simulink model "full_system"  (R2021b)
settings: Solver=FixedStepDiscrete  StartTime=0.0  StopTime=223000  RelTol=1e-3
model workspace (MAT data in the model file):
  out_size = 0
undefined symbols (not defined in the file): betas, bias, DiscIntNeverNeededParam, mus, scale, sigmas
libraries: hdlsllib x1
(part 2 of 3)

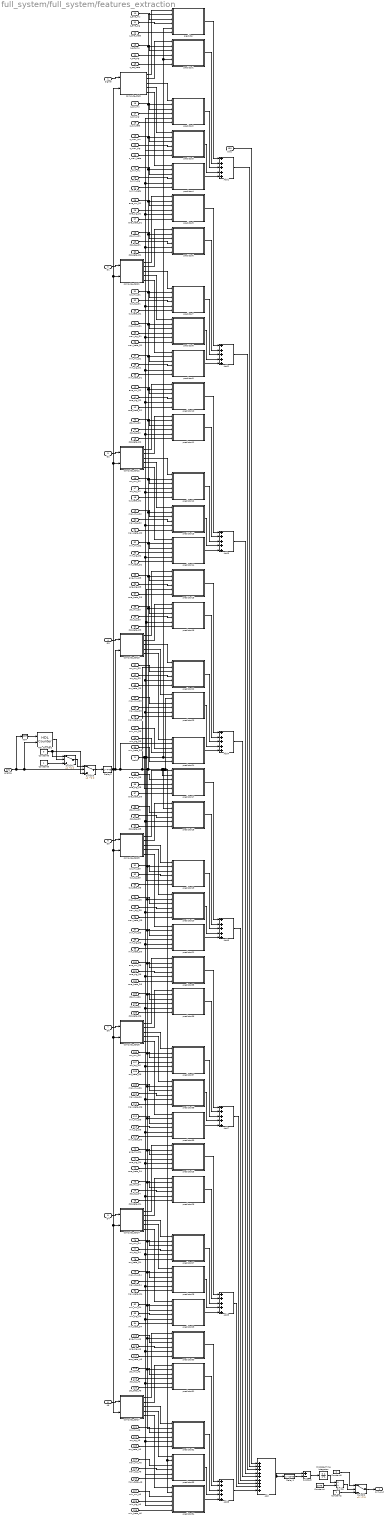
== system full_system/full_system/features_extraction ==
  Signal : Inport
  D1 : Inport  Port=2
  D2 : Inport  Port=3
  D3 : Inport  Port=4
  D4 : Inport  Port=5
  D5 : Inport  Port=6
  D6 : Inport  Port=7
  A6 : Inport  Port=8
  scale : Inport  Port=9
  s_ene_mu : Inport  Port=10
  s_ene_sig : Inport  Port=11
  s_ene_beta : Inport  Port=12
  s_act_mu : Inport  Port=13
  s_act_sig : Inport  Port=14
  s_act_beta : Inport  Port=15
  s_cur_mu : Inport  Port=16
  s_cur_sig : Inport  Port=17
  s_cur_beta : Inport  Port=18
  s_max_mu : Inport  Port=19
  s_max_sig : Inport  Port=20
  s_max_beta : Inport  Port=21
  s_min_mu : Inport  Port=22
  s_min_sig : Inport  Port=23
  s_min_beta : Inport  Port=24
  ene_mu_D1 : Inport  Port=25
  ene_sig_D1 : Inport  Port=26
  ene_beta_D1 : Inport  Port=27
  std_mu_D1 : Inport  Port=28
  std_sig_D1 : Inport  Port=29
  std_beta_D1 : Inport  Port=30
  cur_mu_D1 : Inport  Port=31
  cur_sig_D1 : Inport  Port=32
  cur_beta_D1 : Inport  Port=33
  max_mu_D1 : Inport  Port=34
  max_sig_D1 : Inport  Port=35
  max_beta_D1 : Inport  Port=36
  min_mu_D1 : Inport  Port=37
  min_sig_D1 : Inport  Port=38
  min_beta_D1 : Inport  Port=39
  ene_mu_D2 : Inport  Port=40
  ene_sig_D2 : Inport  Port=41
  ene_beta_D2 : Inport  Port=42
  std_mu_D2 : Inport  Port=43
  std_sig_D2 : Inport  Port=44
  std_beta_D2 : Inport  Port=45
  cur_mu_D2 : Inport  Port=46
  cur_sig_D2 : Inport  Port=47
  cur_beta_D2 : Inport  Port=48
  max_mu_D2 : Inport  Port=49
  max_sig_D2 : Inport  Port=50
  max_beta_D2 : Inport  Port=51
  min_mu_D2 : Inport  Port=52
  min_sig_D2 : Inport  Port=53
  min_beta_D2 : Inport  Port=54
  ene_mu_D3 : Inport  Port=55
  ene_sig_D3 : Inport  Port=56
  ene_beta_D3 : Inport  Port=57
  std_mu_D3 : Inport  Port=58
  std_sig_D3 : Inport  Port=59
  std_beta_D3 : Inport  Port=60
  cur_mu_D3 : Inport  Port=61
  cur_sig_D3 : Inport  Port=62
  cur_beta_D3 : Inport  Port=63
  max_mu_D3 : Inport  Port=64
  max_sig_D3 : Inport  Port=65
  max_beta_D3 : Inport  Port=66
  min_mu_D3 : Inport  Port=67
  min_sig_D3 : Inport  Port=68
  min_beta_D3 : Inport  Port=69
  ene_mu_D4 : Inport  Port=70
  ene_sig_D4 : Inport  Port=71
  ene_beta_D4 : Inport  Port=72
  std_mu_D4 : Inport  Port=73
  std_sig_D4 : Inport  Port=74
  std_beta_D4 : Inport  Port=75
  cur_mu_D4 : Inport  Port=76
  cur_sig_D4 : Inport  Port=77
  cur_beta_D4 : Inport  Port=78
  max_mu_D4 : Inport  Port=79
  max_sig_D4 : Inport  Port=80
  max_beta_D4 : Inport  Port=81
  min_mu_D4 : Inport  Port=82
  min_sig_D4 : Inport  Port=83
  min_beta_D4 : Inport  Port=84
  ene_mu_D5 : Inport  Port=85
  ene_sig_D5 : Inport  Port=86
  ene_beta_D5 : Inport  Port=87
  std_mu_D5 : Inport  Port=88
  std_sig_D5 : Inport  Port=89
  std_beta_D5 : Inport  Port=90
  cur_mu_D5 : Inport  Port=91
  cur_sig_D5 : Inport  Port=92
  cur_beta_D5 : Inport  Port=93
  max_mu_D5 : Inport  Port=94
  max_sig_D5 : Inport  Port=95
  max_beta_D5 : Inport  Port=96
  min_mu_D5 : Inport  Port=97
  min_sig_D5 : Inport  Port=98
  min_beta_D5 : Inport  Port=99
  ene_mu_D6 : Inport  Port=100
  ene_sig_D6 : Inport  Port=101
  ene_beta_D6 : Inport  Port=102
  std_mu_D6 : Inport  Port=103
  std_sig_D6 : Inport  Port=104
  std_beta_D6 : Inport  Port=105
  cur_mu_D6 : Inport  Port=106
  cur_sig_D6 : Inport  Port=107
  cur_beta_D6 : Inport  Port=108
  max_mu_D6 : Inport  Port=109
  max_sig_D6 : Inport  Port=110
  max_beta_D6 : Inport  Port=111
  min_mu_D6 : Inport  Port=112
  min_sig_D6 : Inport  Port=113
  min_beta_D6 : Inport  Port=114
  ene_mu_A6 : Inport  Port=115
  ene_sig_A6 : Inport  Port=116
  ene_beta_A6 : Inport  Port=117
  std_mu_A6 : Inport  Port=118
  std_sig_A6 : Inport  Port=119
  std_beta_A6 : Inport  Port=120
  cur_mu_A6 : Inport  Port=121
  cur_sig_A6 : Inport  Port=122
  cur_beta_A6 : Inport  Port=123
  max_mu_A6 : Inport  Port=124
  max_sig_A6 : Inport  Port=125
  max_beta_A6 : Inport  Port=126
  min_mu_A6 : Inport  Port=127
  min_sig_A6 : Inport  Port=128
  min_beta_A6 : Inport  Port=129
  bias : Inport  Port=130
  enable : Inport  Port=131
  Add : Sum  Inputs=+++++++++
  Add{1..8} (8 alike) : Sum  Inputs=+++++
  Constant2 : Constant  VectorParams1D=off  OutDataTypeStr=uint8  SampleTime=-1
  Constant3 : Constant  Value=0  VectorParams1D=off  OutDataTypeStr=uint8  SampleTime=-1
  Constant4 : Constant  Value=2048  VectorParams1D=off  OutDataTypeStr=uint16  SampleTime=-1
  Constant5 : Constant  VectorParams1D=off  OutDataTypeStr=boolean  SampleTime=-1
  Constant6 : Constant  Value=0  VectorParams1D=off  OutDataTypeStr=boolean  SampleTime=-1
  Delay1 : Delay  DelayLength=2049  InitialCondition=0  UseCircularBuffer=on
  Delay2 : Delay  DelayLength=449  InitialCondition=0  UseCircularBuffer=on
  Discrete-Time Integrator : DiscreteIntegrator  IntegratorMethod=Accumulation: Backward Euler  SampleTime=-1  ICPrevOutput=DiscIntNeverNeededParam  ICPrevScaledInput=DiscIntNeverNeededParam
  Divide : Product  Inputs=*/  RndMeth=Zero  SaturateOnIntegerOverflow=on  OutDataTypeStr=Inherit: Same as first input
  HDL Counter1 : hdlsllib/Sources/HDL Counter  CountType=Count limited  CountInit=0  CountStep=1  CountMax=511  CountFromType=Initial value  CountFrom=0  CountResetPort=on  CountLoadPort=off  CountEnbPort=on  CountDirPort=off  CountHitOutputPort=off  CountDataType=Unsigned  CountWordLen=9  CountFracLen=0  CountSampTime=1
  NOT : Logic  Operator=NOT  IconShape=distinctive  AllPortsSameDT=off  OutDataTypeStr=boolean
  Subtract : Sum  Inputs=+-
  Switch1 : Switch  Criteria=u2 ~= 0
  Switch2 : Switch
  Switch3 : Switch  Criteria=u2 ~= 0
  compute_stats : Subsystem
  compute_stats1 : Subsystem
  compute_stats2 : Subsystem
  compute_stats3 : Subsystem
  compute_stats4 : Subsystem
  compute_stats5 : Subsystem
  compute_stats6 : Subsystem
  compute_stats7 : Subsystem
  predictor{,1..39} (40 alike) : Subsystem  ReferencedSubsystem=predictor_2021b
  svm_out : Outport
  wires:
  cur_sig_D4/1 -> predictor27/4
  predictor1/1 -> Add1/2
  HDL Counter1/1 -> Switch1/2
  ene_mu_D1/1 -> predictor5/3
  Constant5/1 -> Switch1/3
  compute_stats1/1(energy) -> predictor5/1
  predictor11/1 -> Add3/2
  Delay1/1 -> Subtract/2
  compute_stats2/2(std) -> predictor11/1
  predictor29/1 -> Add5/5
  Constant4/1 -> Divide/2
  std_sig_A6/1 -> predictor31/4
  Switch1/1 -> Switch3/1  "trigger"
  predictor3/1 -> Add1/4
  Add1/1 -> Add/2
  Add3/1 -> Add/4
  NOT/1 -> HDL Counter1/1
  s_ene_sig/1 -> predictor/4
  Switch3/1 -> Delay2/1  "trigger"
  compute_stats6/1(energy) -> predictor35/1
  Discrete-Time Integrator/1 -> Divide/1
  compute_stats5/3(curve_l) -> predictor19/1
  predictor13/1 -> Add3/4
  Divide/1 -> Switch2/2  "average"
  predictor18/1 -> Add6/2
  predictor39/1 -> Add7/5
  Switch2/1 -> svm_out/1  "out"
  Subtract/1 -> Discrete-Time Integrator/1
  predictor5/1 -> Add2/1
  predictor23/1 -> Add4/4
  bias/1 -> Add/1
  Add2/1 -> Add/3
  predictor14/1 -> Add3/5
  std_sig_D3/1 -> predictor16/4
  predictor31/1 -> Add8/2
  max_mu_D2/1 -> predictor13/3
  Add4/1 -> Add/5
  std_mu_D2/1 -> predictor11/3
  Add5/1 -> Add/8
  max_mu_D3/1 -> predictor23/3
  predictor32/1 -> Add8/3
  Add6/1 -> Add/6
  Add7/1 -> Add/7
  predictor22/1 -> Add4/3
  Add8/1 -> Add/9
  predictor33/1 -> Add8/4
  ene_sig_A6/1 -> predictor30/4
  predictor6/1 -> Add2/2
  predictor10/1 -> Add3/1
  compute_stats7/2(std) -> predictor31/1
  predictor30/1 -> Add8/1
  predictor34/1 -> Add8/5
  predictor37/1 -> Add7/3
  predictor36/1 -> Add7/2
  predictor38/1 -> Add7/4
  predictor35/1 -> Add7/1
  min_mu_D5/1 -> predictor21/3
  predictor19/1 -> Add6/3
  predictor20/1 -> Add6/4
  max_beta_A6/1 -> predictor33/6
  predictor17/1 -> Add6/1
  compute_stats6/3(curve_l) -> predictor37/1
  predictor21/1 -> Add6/5
  predictor27/1 -> Add5/3
  predictor26/1 -> Add5/2
  predictor28/1 -> Add5/4
  predictor8/1 -> Add2/4
  predictor25/1 -> Add5/1
  predictor16/1 -> Add4/2
  predictor12/1 -> Add3/3
  predictor15/1 -> Add4/1
  Constant2/1 -> Switch2/3
  min_mu_D1/1 -> predictor9/3
  predictor/1 -> Add1/1
  predictor24/1 -> Add4/5
  ene_mu_D2/1 -> predictor10/3
  predictor7/1 -> Add2/3
  predictor9/1 -> Add2/5
  predictor4/1 -> Add1/5
  ene_sig_D4/1 -> predictor25/4
  predictor2/1 -> Add1/3
  min_beta_A6/1 -> predictor34/6
  cur_sig_A6/1 -> predictor32/4
  cur_mu_A6/1 -> predictor32/3
  max_mu_A6/1 -> predictor33/3
  min_mu_A6/1 -> predictor34/3
  std_mu_A6/1 -> predictor31/3
  cur_beta_A6/1 -> predictor32/6
  ene_beta_A6/1 -> predictor30/6
  std_beta_A6/1 -> predictor31/6
  min_sig_A6/1 -> predictor34/4
  ene_mu_A6/1 -> predictor30/3
  max_sig_A6/1 -> predictor33/4
  min_beta_D6/1 -> predictor39/6
  max_beta_D6/1 -> predictor38/6
  cur_sig_D6/1 -> predictor37/4
  cur_mu_D6/1 -> predictor37/3
  max_mu_D6/1 -> predictor38/3
  ene_sig_D6/1 -> predictor35/4
  min_mu_D6/1 -> predictor39/3
  std_sig_D6/1 -> predictor36/4
  std_mu_D6/1 -> predictor36/3
  cur_beta_D6/1 -> predictor37/6
  ene_beta_D6/1 -> predictor35/6
  std_beta_D6/1 -> predictor36/6
  min_sig_D6/1 -> predictor39/4
  ene_mu_D6/1 -> predictor35/3
  max_sig_D6/1 -> predictor38/4
  min_beta_D5/1 -> predictor21/6
  max_beta_D5/1 -> predictor20/6
  cur_sig_D5/1 -> predictor19/4
  cur_mu_D5/1 -> predictor19/3
  max_mu_D5/1 -> predictor20/3
  ene_sig_D5/1 -> predictor17/4
  std_sig_D5/1 -> predictor18/4
  std_mu_D5/1 -> predictor18/3
  cur_beta_D5/1 -> predictor19/6
  ene_beta_D5/1 -> predictor17/6
  std_beta_D5/1 -> predictor18/6
  min_sig_D5/1 -> predictor21/4
  ene_mu_D5/1 -> predictor17/3
  max_sig_D5/1 -> predictor20/4
  min_beta_D4/1 -> predictor29/6
  max_beta_D4/1 -> predictor28/6
  cur_mu_D4/1 -> predictor27/3
  Constant6/1 -> Switch1/1, Switch3/3
  max_mu_D4/1 -> predictor28/3
  min_mu_D4/1 -> predictor29/3
  std_sig_D4/1 -> predictor26/4
  std_mu_D4/1 -> predictor26/3
  cur_beta_D4/1 -> predictor27/6
  ene_beta_D4/1 -> predictor25/6
  std_beta_D4/1 -> predictor26/6
  min_sig_D4/1 -> predictor29/4
  ene_mu_D4/1 -> predictor25/3
  max_sig_D4/1 -> predictor28/4
  min_beta_D3/1 -> predictor24/6
  max_beta_D3/1 -> predictor23/6
  compute_stats5/5(min) -> predictor21/1
  cur_sig_D3/1 -> predictor22/4
  cur_mu_D3/1 -> predictor22/3
  ene_sig_D3/1 -> predictor15/4
  min_mu_D3/1 -> predictor24/3
  std_mu_D3/1 -> predictor16/3
  cur_beta_D3/1 -> predictor22/6
  ene_beta_D3/1 -> predictor15/6
  std_beta_D3/1 -> predictor16/6
  min_sig_D3/1 -> predictor24/4
  compute_stats6/2(std) -> predictor36/1
  ene_mu_D3/1 -> predictor15/3
  max_sig_D3/1 -> predictor23/4
  min_beta_D2/1 -> predictor14/6
  D3/1 -> compute_stats3/1(in)
  max_beta_D2/1 -> predictor13/6
  cur_sig_D2/1 -> predictor12/4
  cur_mu_D2/1 -> predictor12/3
  ene_sig_D2/1 -> predictor10/4
  compute_stats7/1(energy) -> predictor30/1
  min_mu_D2/1 -> predictor14/3
  std_sig_D2/1 -> predictor11/4
  cur_beta_D2/1 -> predictor12/6
  ene_beta_D2/1 -> predictor10/6
  std_beta_D2/1 -> predictor11/6
  min_sig_D2/1 -> predictor14/4
  max_sig_D2/1 -> predictor13/4
  min_beta_D1/1 -> predictor9/6
  max_beta_D1/1 -> predictor8/6
  cur_sig_D1/1 -> predictor7/4
  cur_mu_D1/1 -> predictor7/3
  max_mu_D1/1 -> predictor8/3
  ene_sig_D1/1 -> predictor5/4
  std_sig_D1/1 -> predictor6/4
  std_mu_D1/1 -> predictor6/3
  cur_beta_D1/1 -> predictor7/6
  ene_beta_D1/1 -> predictor5/6
  std_beta_D1/1 -> predictor6/6
  min_sig_D1/1 -> predictor9/4
  max_sig_D1/1 -> predictor8/4
  s_min_beta/1 -> predictor4/6
  s_min_mu/1 -> predictor4/3
  s_min_sig/1 -> predictor4/4
  s_max_beta/1 -> predictor3/6
  s_max_mu/1 -> predictor3/3
  s_max_sig/1 -> predictor3/4
  s_cur_beta/1 -> predictor2/6
  s_cur_mu/1 -> predictor2/3
  s_cur_sig/1 -> predictor2/4
  s_act_beta/1 -> predictor1/6
  s_act_mu/1 -> predictor1/3
  s_act_sig/1 -> predictor1/4
  s_ene_beta/1 -> predictor/6
  s_ene_mu/1 -> predictor/3
  compute_stats3/5(min) -> predictor24/1
  compute_stats7/5(min) -> predictor34/1
  compute_stats7/4(max) -> predictor33/1
  compute_stats7/3(curve_l) -> predictor32/1
  Delay2/1 -> compute_stats7/2(trigger), compute_stats4/2(trigger), compute_stats6/2(trigger), compute_stats5/2(trigger), predictor32/2, predictor31/2, predictor30/2, predictor29/2, predictor28/2, predictor27/2, predictor26/2, predictor25/2, predictor39/2, predictor38/2, predictor37/2, predictor36/2, predictor35/2, predictor21/2, predictor20/2, predictor19/2, predictor33/2, predictor34/2, predictor23/2, predictor18/2, predictor17/2, predictor1/2, predictor/2, predictor2/2, predictor3/2, predictor4/2, predictor5/2, predictor6/2, predictor7/2, predictor8/2, predictor9/2, predictor10/2, predictor11/2, predictor12/2, predictor13/2, predictor14/2, predictor15/2, predictor16/2, predictor22/2, predictor24/2, compute_stats3/2(trigger), compute_stats1/2(trigger), compute_stats/2(trigger), compute_stats2/2(trigger)  "trigger"
  compute_stats6/5(min) -> predictor39/1
  compute_stats6/4(max) -> predictor38/1
  compute_stats5/4(max) -> predictor20/1
  compute_stats5/2(std) -> predictor18/1
  compute_stats5/1(energy) -> predictor17/1
  compute_stats4/5(min) -> predictor29/1
  compute_stats4/4(max) -> predictor28/1
  compute_stats4/3(curve_l) -> predictor27/1
  compute_stats4/2(std) -> predictor26/1
  compute_stats4/1(energy) -> predictor25/1
  compute_stats3/4(max) -> predictor23/1
  compute_stats3/3(curve_l) -> predictor22/1
  compute_stats3/2(std) -> predictor16/1
  compute_stats3/1(energy) -> predictor15/1
  compute_stats2/5(min) -> predictor14/1
  compute_stats2/4(max) -> predictor13/1
  compute_stats2/3(curve_l) -> predictor12/1
  compute_stats2/1(energy) -> predictor10/1
  compute_stats1/5(min) -> predictor9/1
  compute_stats1/4(max) -> predictor8/1
  compute_stats1/3(curve_l) -> predictor7/1
  compute_stats1/2(std) -> predictor6/1
  compute_stats/5(min) -> predictor4/1
  compute_stats/4(max) -> predictor3/1
  compute_stats/3(curve_l) -> predictor2/1
  compute_stats/2(activity) -> predictor1/1
  compute_stats/1(energy) -> predictor/1
  Add/1 -> Delay1/1, Subtract/1  "in"
  Constant3/1 -> Switch2/1
  A6/1 -> compute_stats7/1(in)
  D6/1 -> compute_stats6/1(in)
  D5/1 -> compute_stats5/1(in)
  D4/1 -> compute_stats4/1(in)
  D2/1 -> compute_stats2/1(in)
  D1/1 -> compute_stats1/1(in)
  Signal/1 -> compute_stats/1(in)  "signal"
  enable/1 -> HDL Counter1/2, Switch3/2, NOT/1
  scale/1 -> predictor34/5, predictor32/5, predictor31/5, predictor30/5, predictor29/5, predictor28/5, predictor27/5, predictor26/5, predictor25/5, predictor33/5, predictor39/5, predictor38/5, predictor37/5, predictor36/5, predictor35/5, predictor21/5, predictor20/5, predictor18/5, predictor1/5, predictor/5, predictor24/5, predictor16/5, predictor15/5, predictor19/5, predictor4/5, predictor3/5, predictor5/5, predictor6/5, predictor7/5, predictor8/5, predictor9/5, predictor10/5, predictor11/5, predictor12/5, predictor13/5, predictor14/5, predictor22/5, predictor23/5, predictor2/5, predictor17/5

== system full_system/full_system/4_level_dwt/1_level_dwt ==
  s_in : Inport
  enable : Inport  Port=2
  Constant : Constant  Value=0  OutDataTypeStr=Inherit: Inherit via back propagation  SampleTime=-1
  Discrete FIR Filter : DiscreteFir  CoefSource=Input port
      settings: InputPortMap=u0,u1
  Discrete FIR Filter1 : DiscreteFir  CoefSource=Input port
      settings: InputPortMap=u0,u1
  Downsample : DownSample  phase=1  RateOptions=Allow multirate processing
  Downsample1 : DownSample  phase=1  RateOptions=Allow multirate processing
  RT2 : RateTransition  OutPortSampleTime=2
  Switch : Switch  Criteria=u2 > Threshold
  Switch1 : Switch  Criteria=u2 > Threshold
  db4 scaling : Constant  Value="[-0.0106    0.0329    0.0308   -0.1870   -0.0280    0.6309    0.7148    0.2304]"  OutDataTypeStr=Inherit: Inherit via back propagation  SampleTime=-1
  db4 wavelet : Constant  Value="[-0.2304    0.7148   -0.6309   -0.0280    0.1870    0.0308   -0.0329   -0.0106]"  OutDataTypeStr=Inherit: Inherit via back propagation  SampleTime=-1
  D : Outport
  A : Outport  Port=2
  wires:
  db4 wavelet/1 -> Discrete FIR Filter/2
  s_in/1 -> Discrete FIR Filter1/1, Discrete FIR Filter/1
  db4 scaling/1 -> Discrete FIR Filter1/2
  Constant/1 -> Switch/3, Switch1/3
  Discrete FIR Filter/1 -> Downsample/1
  Discrete FIR Filter1/1 -> Downsample1/1
  Switch1/1 -> A/1
  Switch/1 -> D/1
  Downsample/1 -> Switch/1
  Downsample1/1 -> Switch1/1
  enable/1 -> RT2/1
  RT2/1 -> Switch/2, Switch1/2

== system full_system/full_system/4_level_dwt/1_level_dwt1 ==
  s_in : Inport
  enable : Inport  Port=2
  Constant : Constant  Value=0  OutDataTypeStr=Inherit: Inherit via back propagation  SampleTime=-1
  Discrete FIR Filter : DiscreteFir  CoefSource=Input port
      settings: InputPortMap=u0,u1
  Discrete FIR Filter1 : DiscreteFir  CoefSource=Input port
      settings: InputPortMap=u0,u1
  Downsample : DownSample  phase=1  RateOptions=Allow multirate processing
  Downsample1 : DownSample  phase=1  RateOptions=Allow multirate processing
  RT2 : RateTransition  OutPortSampleTime=4
  Switch : Switch  Criteria=u2 > Threshold
  Switch1 : Switch  Criteria=u2 > Threshold
  db4 scaling : Constant  Value="[-0.0106    0.0329    0.0308   -0.1870   -0.0280    0.6309    0.7148    0.2304]"  OutDataTypeStr=Inherit: Inherit via back propagation  SampleTime=-1
  db4 wavelet : Constant  Value="[-0.2304    0.7148   -0.6309   -0.0280    0.1870    0.0308   -0.0329   -0.0106]"  OutDataTypeStr=Inherit: Inherit via back propagation  SampleTime=-1
  D : Outport
  A : Outport  Port=2
  wires:
  db4 wavelet/1 -> Discrete FIR Filter/2
  s_in/1 -> Discrete FIR Filter1/1, Discrete FIR Filter/1
  db4 scaling/1 -> Discrete FIR Filter1/2
  Constant/1 -> Switch/3, Switch1/3
  Discrete FIR Filter/1 -> Downsample/1
  Discrete FIR Filter1/1 -> Downsample1/1
  Switch1/1 -> A/1
  Switch/1 -> D/1
  Downsample/1 -> Switch/1
  Downsample1/1 -> Switch1/1
  enable/1 -> RT2/1
  RT2/1 -> Switch/2, Switch1/2

== system full_system/full_system/4_level_dwt/1_level_dwt2 ==
  s_in : Inport
  enable : Inport  Port=2
  Constant : Constant  Value=0  OutDataTypeStr=Inherit: Inherit via back propagation  SampleTime=-1
  Discrete FIR Filter : DiscreteFir  CoefSource=Input port
      settings: InputPortMap=u0,u1
  Discrete FIR Filter1 : DiscreteFir  CoefSource=Input port
      settings: InputPortMap=u0,u1
  Downsample : DownSample  phase=1  RateOptions=Allow multirate processing
  Downsample1 : DownSample  phase=1  RateOptions=Allow multirate processing
  RT2 : RateTransition  OutPortSampleTime=8
  Switch : Switch  Criteria=u2 > Threshold
  Switch1 : Switch  Criteria=u2 > Threshold
  db4 scaling : Constant  Value="[-0.0106    0.0329    0.0308   -0.1870   -0.0280    0.6309    0.7148    0.2304]"  OutDataTypeStr=Inherit: Inherit via back propagation  SampleTime=-1
  db4 wavelet : Constant  Value="[-0.2304    0.7148   -0.6309   -0.0280    0.1870    0.0308   -0.0329   -0.0106]"  OutDataTypeStr=Inherit: Inherit via back propagation  SampleTime=-1
  D : Outport
  A : Outport  Port=2
  wires:
  db4 wavelet/1 -> Discrete FIR Filter/2
  s_in/1 -> Discrete FIR Filter1/1, Discrete FIR Filter/1
  db4 scaling/1 -> Discrete FIR Filter1/2
  Constant/1 -> Switch/3, Switch1/3
  Discrete FIR Filter/1 -> Downsample/1
  Discrete FIR Filter1/1 -> Downsample1/1
  Switch1/1 -> A/1
  Switch/1 -> D/1
  Downsample/1 -> Switch/1
  Downsample1/1 -> Switch1/1
  enable/1 -> RT2/1
  RT2/1 -> Switch/2, Switch1/2

== system full_system/full_system/4_level_dwt/1_level_dwt3 ==
  s_in : Inport
  enable : Inport  Port=2
  Constant : Constant  Value=0  OutDataTypeStr=Inherit: Inherit via back propagation  SampleTime=-1
  Discrete FIR Filter : DiscreteFir  CoefSource=Input port
      settings: InputPortMap=u0,u1
  Discrete FIR Filter1 : DiscreteFir  CoefSource=Input port
      settings: InputPortMap=u0,u1
  Downsample : DownSample  phase=1  RateOptions=Allow multirate processing
  Downsample1 : DownSample  phase=1  RateOptions=Allow multirate processing
  RT2 : RateTransition  OutPortSampleTime=16
  Switch : Switch  Criteria=u2 > Threshold
  Switch1 : Switch  Criteria=u2 > Threshold
  db4 scaling : Constant  Value="[-0.0106    0.0329    0.0308   -0.1870   -0.0280    0.6309    0.7148    0.2304]"  OutDataTypeStr=Inherit: Inherit via back propagation  SampleTime=-1
  db4 wavelet : Constant  Value="[-0.2304    0.7148   -0.6309   -0.0280    0.1870    0.0308   -0.0329   -0.0106]"  OutDataTypeStr=Inherit: Inherit via back propagation  SampleTime=-1
  D : Outport
  A : Outport  Port=2
  wires:
  db4 wavelet/1 -> Discrete FIR Filter/2
  s_in/1 -> Discrete FIR Filter1/1, Discrete FIR Filter/1
  db4 scaling/1 -> Discrete FIR Filter1/2
  Constant/1 -> Switch/3, Switch1/3
  Discrete FIR Filter/1 -> Downsample/1
  Switch1/1 -> A/1
  Switch/1 -> D/1
  Downsample/1 -> Switch/1
  Downsample1/1 -> Switch1/1
  enable/1 -> RT2/1
  RT2/1 -> Switch/2, Switch1/2
  Discrete FIR Filter1/1 -> Downsample1/1

== system full_system/full_system/4_level_dwt/1_level_dwt4 ==
  s_in : Inport
  enable : Inport  Port=2
  Constant : Constant  Value=0  OutDataTypeStr=Inherit: Inherit via back propagation  SampleTime=-1
  Discrete FIR Filter : DiscreteFir  CoefSource=Input port
      settings: InputPortMap=u0,u1
  Discrete FIR Filter1 : DiscreteFir  CoefSource=Input port
      settings: InputPortMap=u0,u1
  Downsample : DownSample  phase=1  RateOptions=Allow multirate processing
  Downsample1 : DownSample  phase=1  RateOptions=Allow multirate processing
  RT2 : RateTransition  OutPortSampleTime=32
  Switch : Switch  Criteria=u2 > Threshold
  Switch1 : Switch  Criteria=u2 > Threshold
  db4 scaling : Constant  Value="[-0.0106    0.0329    0.0308   -0.1870   -0.0280    0.6309    0.7148    0.2304]"  OutDataTypeStr=Inherit: Inherit via back propagation  SampleTime=-1
  db4 wavelet : Constant  Value="[-0.2304    0.7148   -0.6309   -0.0280    0.1870    0.0308   -0.0329   -0.0106]"  OutDataTypeStr=Inherit: Inherit via back propagation  SampleTime=-1
  D : Outport
  A : Outport  Port=2
  wires:
  db4 wavelet/1 -> Discrete FIR Filter/2
  s_in/1 -> Discrete FIR Filter1/1, Discrete FIR Filter/1
  db4 scaling/1 -> Discrete FIR Filter1/2
  Constant/1 -> Switch/3, Switch1/3
  Discrete FIR Filter/1 -> Downsample/1
  Switch1/1 -> A/1
  Switch/1 -> D/1
  Downsample/1 -> Switch/1
  Downsample1/1 -> Switch1/1
  enable/1 -> RT2/1
  RT2/1 -> Switch/2, Switch1/2
  Discrete FIR Filter1/1 -> Downsample1/1

== system full_system/full_system/4_level_dwt/1_level_dwt5 ==
  s_in : Inport
  enable : Inport  Port=2
  Constant : Constant  Value=0  OutDataTypeStr=Inherit: Inherit via back propagation  SampleTime=-1
  Discrete FIR Filter : DiscreteFir  CoefSource=Input port
      settings: InputPortMap=u0,u1
  Discrete FIR Filter1 : DiscreteFir  CoefSource=Input port
      settings: InputPortMap=u0,u1
  Downsample : DownSample  phase=1  RateOptions=Allow multirate processing
  Downsample1 : DownSample  phase=1  RateOptions=Allow multirate processing
  RT2 : RateTransition  OutPortSampleTime=64
  Switch : Switch  Criteria=u2 > Threshold
  Switch1 : Switch  Criteria=u2 > Threshold
  db4 scaling : Constant  Value="[-0.0106    0.0329    0.0308   -0.1870   -0.0280    0.6309    0.7148    0.2304]"  OutDataTypeStr=Inherit: Inherit via back propagation  SampleTime=-1
  db4 wavelet : Constant  Value="[-0.2304    0.7148   -0.6309   -0.0280    0.1870    0.0308   -0.0329   -0.0106]"  OutDataTypeStr=Inherit: Inherit via back propagation  SampleTime=-1
  D : Outport
  A : Outport  Port=2
  wires:
  db4 wavelet/1 -> Discrete FIR Filter/2
  s_in/1 -> Discrete FIR Filter1/1, Discrete FIR Filter/1
  db4 scaling/1 -> Discrete FIR Filter1/2
  Constant/1 -> Switch/3, Switch1/3
  Discrete FIR Filter/1 -> Downsample/1
  Switch1/1 -> A/1
  Switch/1 -> D/1
  Downsample/1 -> Switch/1
  Downsample1/1 -> Switch1/1
  enable/1 -> RT2/1
  RT2/1 -> Switch/2, Switch1/2
  Discrete FIR Filter1/1 -> Downsample1/1

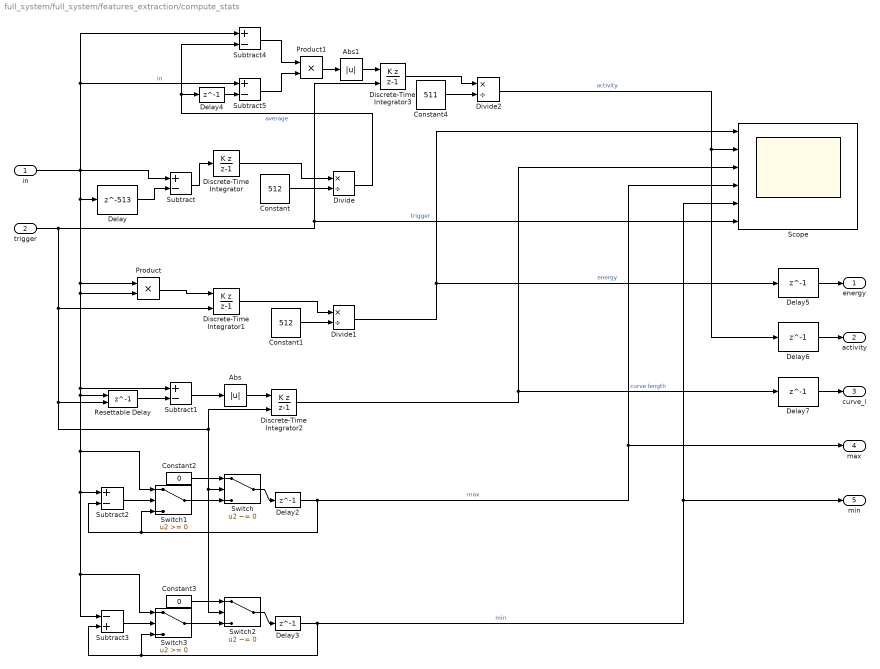
== system full_system/full_system/features_extraction/compute_stats ==
  in : Inport
  trigger : Inport  Port=2
  Abs : Abs
  Abs1 : Abs
  Constant : Constant  Value=512  VectorParams1D=off  OutDataTypeStr=uint16  SampleTime=-1
  Constant1 : Constant  Value=512  VectorParams1D=off  OutDataTypeStr=uint16  SampleTime=-1
  Constant2 : Constant  Value=0  VectorParams1D=off  OutDataTypeStr=uint8  SampleTime=-1
  Constant3 : Constant  Value=0  VectorParams1D=off  OutDataTypeStr=uint8  SampleTime=-1
  Constant4 : Constant  Value=511  VectorParams1D=off  OutDataTypeStr=uint16  SampleTime=-1
  Delay : Delay  DelayLength=513  InitialCondition=0  UseCircularBuffer=on
  Delay{2..7} (6 alike) : Delay  DelayLength=1  InitialCondition=0  UseCircularBuffer=on
  Discrete-Time Integrator : DiscreteIntegrator  IntegratorMethod=Accumulation: Backward Euler  SampleTime=-1  ICPrevOutput=DiscIntNeverNeededParam  ICPrevScaledInput=DiscIntNeverNeededParam
  Discrete-Time Integrator1 : DiscreteIntegrator  IntegratorMethod=Accumulation: Backward Euler  ExternalReset=rising  SampleTime=-1  ICPrevOutput=DiscIntNeverNeededParam  ICPrevScaledInput=DiscIntNeverNeededParam
  Discrete-Time Integrator2 : DiscreteIntegrator  IntegratorMethod=Accumulation: Backward Euler  ExternalReset=rising  SampleTime=-1  ICPrevOutput=DiscIntNeverNeededParam  ICPrevScaledInput=DiscIntNeverNeededParam
  Discrete-Time Integrator3 : DiscreteIntegrator  IntegratorMethod=Accumulation: Backward Euler  ExternalReset=rising  SampleTime=-1  ICPrevOutput=DiscIntNeverNeededParam  ICPrevScaledInput=DiscIntNeverNeededParam
  Divide : Product  Inputs=*/  RndMeth=Zero  SaturateOnIntegerOverflow=on  OutDataTypeStr=Inherit: Same as first input
  Divide1 : Product  Inputs=*/  RndMeth=Zero  SaturateOnIntegerOverflow=on
  Divide2 : Product  Inputs=*/  RndMeth=Zero  SaturateOnIntegerOverflow=on
  Product : Product
  Product1 : Product
  Resettable Delay : Delay  DelayLength=1  ExternalReset=Level
      settings: InputPortMap=u0,r5
  Scope : Scope  NumInputPorts=6
  Subtract{,1..2,4..5} (5 alike) : Sum  Inputs=+-
  Subtract3 : Sum  Inputs=-+
  Switch : Switch  Criteria=u2 ~= 0
  Switch1 : Switch  OutDataTypeStr=Inherit: Same as first input
  Switch2 : Switch  Criteria=u2 ~= 0
  Switch3 : Switch  OutDataTypeStr=Inherit: Same as first input
  energy : Outport
  activity : Outport  Port=2
  curve_l : Outport  Port=3
  max : Outport  Port=4
  min : Outport  Port=5
  wires:
  Constant/1 -> Divide/2
  Subtract/1 -> Discrete-Time Integrator/1
  Delay/1 -> Subtract/2
  Product/1 -> Discrete-Time Integrator1/1
  Constant1/1 -> Divide1/2
  Discrete-Time Integrator1/1 -> Divide1/1
  Resettable Delay/1 -> Subtract1/2
  Subtract1/1 -> Abs/1
  Abs/1 -> Discrete-Time Integrator2/1
  Discrete-Time Integrator2/1 -> Delay7/1, Scope/3  "curve length"
  Constant2/1 -> Switch/1
  Subtract2/1 -> Switch1/2
  Delay2/1 -> max/1, Scope/4, Switch1/3, Subtract2/2  "max"
  Switch/1 -> Delay2/1
  Switch1/1 -> Switch/3
  Constant3/1 -> Switch2/1
  Switch2/1 -> Delay3/1
  Switch3/1 -> Switch2/3
  Subtract3/1 -> Switch3/2
  Delay3/1 -> min/1, Scope/5, Switch3/3, Subtract3/2  "min"
  Delay4/1 -> Subtract5/2
  Subtract4/1 -> Product1/1
  Subtract5/1 -> Product1/2
  Constant4/1 -> Divide2/2
  Discrete-Time Integrator3/1 -> Divide2/1
  Divide/1 -> Subtract4/2, Delay4/1  "average"
  Discrete-Time Integrator/1 -> Divide/1
  Divide2/1 -> Scope/2, Delay6/1  "activity"
  Product1/1 -> Abs1/1
  Abs1/1 -> Discrete-Time Integrator3/1
  Delay5/1 -> energy/1
  Delay6/1 -> activity/1
  Delay7/1 -> curve_l/1
  Divide1/1 -> Scope/1, Delay5/1  "energy"
  in/1 -> Delay/1, Product/1, Resettable Delay/1, Switch1/1, Switch3/1, Subtract3/1, Subtract2/1, Subtract1/1, Product/2, Subtract4/1, Subtract5/1, Subtract/1  "in"
  trigger/1 -> Discrete-Time Integrator3/2, Scope/6, Discrete-Time Integrator1/2, Resettable Delay/2, Discrete-Time Integrator2/2, Switch2/2, Switch/2  "trigger"

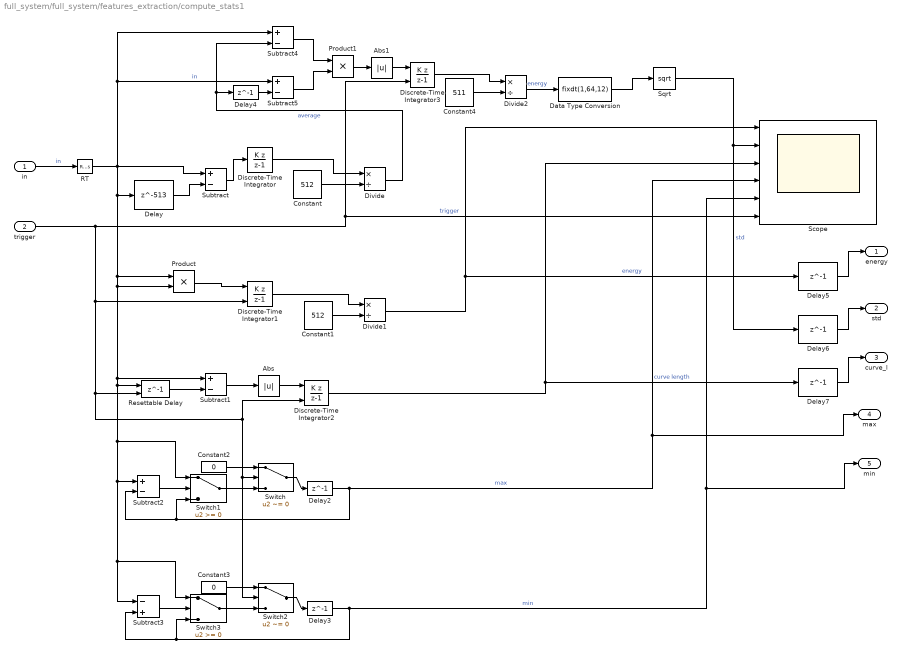
== system full_system/full_system/features_extraction/compute_stats1 ==
  in : Inport
  trigger : Inport  Port=2
  Abs : Abs
  Abs1 : Abs
  Constant : Constant  Value=512  VectorParams1D=off  OutDataTypeStr=uint16  SampleTime=-1
  Constant1 : Constant  Value=512  VectorParams1D=off  OutDataTypeStr=uint16  SampleTime=-1
  Constant2 : Constant  Value=0  VectorParams1D=off  OutDataTypeStr=uint8  SampleTime=-1
  Constant3 : Constant  Value=0  VectorParams1D=off  OutDataTypeStr=uint8  SampleTime=-1
  Constant4 : Constant  Value=511  VectorParams1D=off  OutDataTypeStr=uint16  SampleTime=-1
  Data Type Conversion : DataTypeConversion  OutMax=2  OutDataTypeStr=fixdt(1,64,12)
  Delay : Delay  DelayLength=513  InitialCondition=0  UseCircularBuffer=on
  Delay{2..7} (6 alike) : Delay  DelayLength=1  InitialCondition=0  UseCircularBuffer=on
  Discrete-Time Integrator : DiscreteIntegrator  IntegratorMethod=Accumulation: Backward Euler  SampleTime=-1  ICPrevOutput=DiscIntNeverNeededParam  ICPrevScaledInput=DiscIntNeverNeededParam
  Discrete-Time Integrator1 : DiscreteIntegrator  IntegratorMethod=Accumulation: Backward Euler  ExternalReset=rising  SampleTime=-1  ICPrevOutput=DiscIntNeverNeededParam  ICPrevScaledInput=DiscIntNeverNeededParam
  Discrete-Time Integrator2 : DiscreteIntegrator  IntegratorMethod=Accumulation: Backward Euler  ExternalReset=rising  SampleTime=-1  ICPrevOutput=DiscIntNeverNeededParam  ICPrevScaledInput=DiscIntNeverNeededParam
  Discrete-Time Integrator3 : DiscreteIntegrator  IntegratorMethod=Accumulation: Backward Euler  ExternalReset=rising  SampleTime=-1  ICPrevOutput=DiscIntNeverNeededParam  ICPrevScaledInput=DiscIntNeverNeededParam
  Divide : Product  Inputs=*/  RndMeth=Zero  SaturateOnIntegerOverflow=on  OutDataTypeStr=Inherit: Same as first input
  Divide1 : Product  Inputs=*/  RndMeth=Zero  SaturateOnIntegerOverflow=on
  Divide2 : Product  Inputs=*/  RndMeth=Zero  SaturateOnIntegerOverflow=on
  Product : Product
  Product1 : Product
  RT : RateTransition  OutPortSampleTime=1
  Resettable Delay : Delay  DelayLength=1  ExternalReset=Level
      settings: InputPortMap=u0,r5
  Scope : Scope  NumInputPorts=6
  Sqrt : Sqrt  SaturateOnIntegerOverflow=on
  Subtract{,1..2,4..5} (5 alike) : Sum  Inputs=+-
  Subtract3 : Sum  Inputs=-+
  Switch : Switch  Criteria=u2 ~= 0
  Switch1 : Switch  OutDataTypeStr=Inherit: Same as first input
  Switch2 : Switch  Criteria=u2 ~= 0
  Switch3 : Switch  OutDataTypeStr=Inherit: Same as first input
  energy : Outport
  std : Outport  Port=2
  curve_l : Outport  Port=3
  max : Outport  Port=4
  min : Outport  Port=5
  wires:
  Constant/1 -> Divide/2
  Subtract/1 -> Discrete-Time Integrator/1
  Delay/1 -> Subtract/2
  Product/1 -> Discrete-Time Integrator1/1
  Constant1/1 -> Divide1/2
  Discrete-Time Integrator1/1 -> Divide1/1
  Resettable Delay/1 -> Subtract1/2
  Subtract1/1 -> Abs/1
  Abs/1 -> Discrete-Time Integrator2/1
  Discrete-Time Integrator2/1 -> Delay7/1, Scope/3  "curve length"
  Constant2/1 -> Switch/1
  Subtract2/1 -> Switch1/2
  Delay2/1 -> max/1, Scope/4, Switch1/3, Subtract2/2  "max"
  Switch/1 -> Delay2/1
  Switch1/1 -> Switch/3
  Constant3/1 -> Switch2/1
  Switch2/1 -> Delay3/1
  Switch3/1 -> Switch2/3
  Subtract3/1 -> Switch3/2
  Delay3/1 -> min/1, Scope/5, Switch3/3, Subtract3/2  "min"
  trigger/1 -> Discrete-Time Integrator3/2, Scope/6, Discrete-Time Integrator1/2, Resettable Delay/2, Discrete-Time Integrator2/2, Switch2/2, Switch/2  "trigger"
  RT/1 -> Subtract4/1, Subtract5/1, Delay/1, Product/1, Switch1/1, Switch3/1, Subtract3/1, Subtract2/1, Resettable Delay/1, Subtract1/1, Product/2, Subtract/1  "in"
  Delay4/1 -> Subtract5/2
  Subtract4/1 -> Product1/1
  Subtract5/1 -> Product1/2
  Constant4/1 -> Divide2/2
  Discrete-Time Integrator3/1 -> Divide2/1
  Divide/1 -> Subtract4/2, Delay4/1  "average"
  Discrete-Time Integrator/1 -> Divide/1
  Divide2/1 -> Data Type Conversion/1  "energy"
  Data Type Conversion/1 -> Sqrt/1
  Product1/1 -> Abs1/1
  Abs1/1 -> Discrete-Time Integrator3/1
  Delay5/1 -> energy/1
  Delay6/1 -> std/1
  Delay7/1 -> curve_l/1
  Divide1/1 -> Scope/1, Delay5/1  "energy"
  Sqrt/1 -> Scope/2, Delay6/1  "std"
  in/1 -> RT/1  "in"

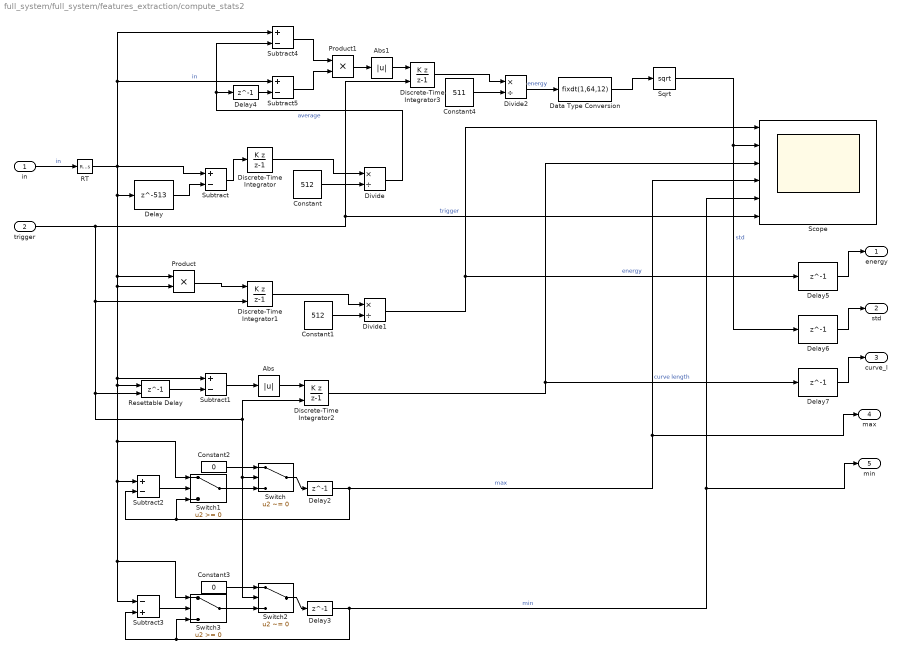
== system full_system/full_system/features_extraction/compute_stats2 ==
  in : Inport
  trigger : Inport  Port=2
  Abs : Abs
  Abs1 : Abs
  Constant : Constant  Value=512  VectorParams1D=off  OutDataTypeStr=uint16  SampleTime=-1
  Constant1 : Constant  Value=512  VectorParams1D=off  OutDataTypeStr=uint16  SampleTime=-1
  Constant2 : Constant  Value=0  VectorParams1D=off  OutDataTypeStr=uint8  SampleTime=-1
  Constant3 : Constant  Value=0  VectorParams1D=off  OutDataTypeStr=uint8  SampleTime=-1
  Constant4 : Constant  Value=511  VectorParams1D=off  OutDataTypeStr=uint16  SampleTime=-1
  Data Type Conversion : DataTypeConversion  OutMax=2  OutDataTypeStr=fixdt(1,64,12)
  Delay : Delay  DelayLength=513  InitialCondition=0  UseCircularBuffer=on
  Delay{2..7} (6 alike) : Delay  DelayLength=1  InitialCondition=0  UseCircularBuffer=on
  Discrete-Time Integrator : DiscreteIntegrator  IntegratorMethod=Accumulation: Backward Euler  SampleTime=-1  ICPrevOutput=DiscIntNeverNeededParam  ICPrevScaledInput=DiscIntNeverNeededParam
  Discrete-Time Integrator1 : DiscreteIntegrator  IntegratorMethod=Accumulation: Backward Euler  ExternalReset=rising  SampleTime=-1  ICPrevOutput=DiscIntNeverNeededParam  ICPrevScaledInput=DiscIntNeverNeededParam
  Discrete-Time Integrator2 : DiscreteIntegrator  IntegratorMethod=Accumulation: Backward Euler  ExternalReset=rising  SampleTime=-1  ICPrevOutput=DiscIntNeverNeededParam  ICPrevScaledInput=DiscIntNeverNeededParam
  Discrete-Time Integrator3 : DiscreteIntegrator  IntegratorMethod=Accumulation: Backward Euler  ExternalReset=rising  SampleTime=-1  ICPrevOutput=DiscIntNeverNeededParam  ICPrevScaledInput=DiscIntNeverNeededParam
  Divide : Product  Inputs=*/  RndMeth=Zero  SaturateOnIntegerOverflow=on  OutDataTypeStr=Inherit: Same as first input
  Divide1 : Product  Inputs=*/  RndMeth=Zero  SaturateOnIntegerOverflow=on
  Divide2 : Product  Inputs=*/  RndMeth=Zero  SaturateOnIntegerOverflow=on
  Product : Product
  Product1 : Product
  RT : RateTransition  OutPortSampleTime=1
  Resettable Delay : Delay  DelayLength=1  ExternalReset=Level
      settings: InputPortMap=u0,r5
  Scope : Scope  NumInputPorts=6
  Sqrt : Sqrt  SaturateOnIntegerOverflow=on
  Subtract{,1..2,4..5} (5 alike) : Sum  Inputs=+-
  Subtract3 : Sum  Inputs=-+
  Switch : Switch  Criteria=u2 ~= 0
  Switch1 : Switch  OutDataTypeStr=Inherit: Same as first input
  Switch2 : Switch  Criteria=u2 ~= 0
  Switch3 : Switch  OutDataTypeStr=Inherit: Same as first input
  energy : Outport
  std : Outport  Port=2
  curve_l : Outport  Port=3
  max : Outport  Port=4
  min : Outport  Port=5
  wires:
  Constant/1 -> Divide/2
  Subtract/1 -> Discrete-Time Integrator/1
  Delay/1 -> Subtract/2
  Product/1 -> Discrete-Time Integrator1/1
  Constant1/1 -> Divide1/2
  Discrete-Time Integrator1/1 -> Divide1/1
  Resettable Delay/1 -> Subtract1/2
  Subtract1/1 -> Abs/1
  Abs/1 -> Discrete-Time Integrator2/1
  Discrete-Time Integrator2/1 -> Delay7/1, Scope/3  "curve length"
  Constant2/1 -> Switch/1
  Subtract2/1 -> Switch1/2
  Delay2/1 -> max/1, Scope/4, Switch1/3, Subtract2/2  "max"
  Switch/1 -> Delay2/1
  Switch1/1 -> Switch/3
  Constant3/1 -> Switch2/1
  Switch2/1 -> Delay3/1
  Switch3/1 -> Switch2/3
  Subtract3/1 -> Switch3/2
  Delay3/1 -> min/1, Scope/5, Switch3/3, Subtract3/2  "min"
  trigger/1 -> Discrete-Time Integrator3/2, Scope/6, Discrete-Time Integrator1/2, Resettable Delay/2, Discrete-Time Integrator2/2, Switch2/2, Switch/2  "trigger"
  RT/1 -> Subtract4/1, Subtract5/1, Delay/1, Product/1, Switch1/1, Switch3/1, Subtract3/1, Subtract2/1, Resettable Delay/1, Subtract1/1, Product/2, Subtract/1  "in"
  Delay4/1 -> Subtract5/2
  Subtract4/1 -> Product1/1
  Subtract5/1 -> Product1/2
  Constant4/1 -> Divide2/2
  Discrete-Time Integrator3/1 -> Divide2/1
  Divide/1 -> Subtract4/2, Delay4/1  "average"
  Discrete-Time Integrator/1 -> Divide/1
  Divide2/1 -> Data Type Conversion/1  "energy"
  Data Type Conversion/1 -> Sqrt/1
  Product1/1 -> Abs1/1
  Abs1/1 -> Discrete-Time Integrator3/1
  Delay5/1 -> energy/1
  Delay6/1 -> std/1
  Delay7/1 -> curve_l/1
  Divide1/1 -> Scope/1, Delay5/1  "energy"
  Sqrt/1 -> Scope/2, Delay6/1  "std"
  in/1 -> RT/1  "in"

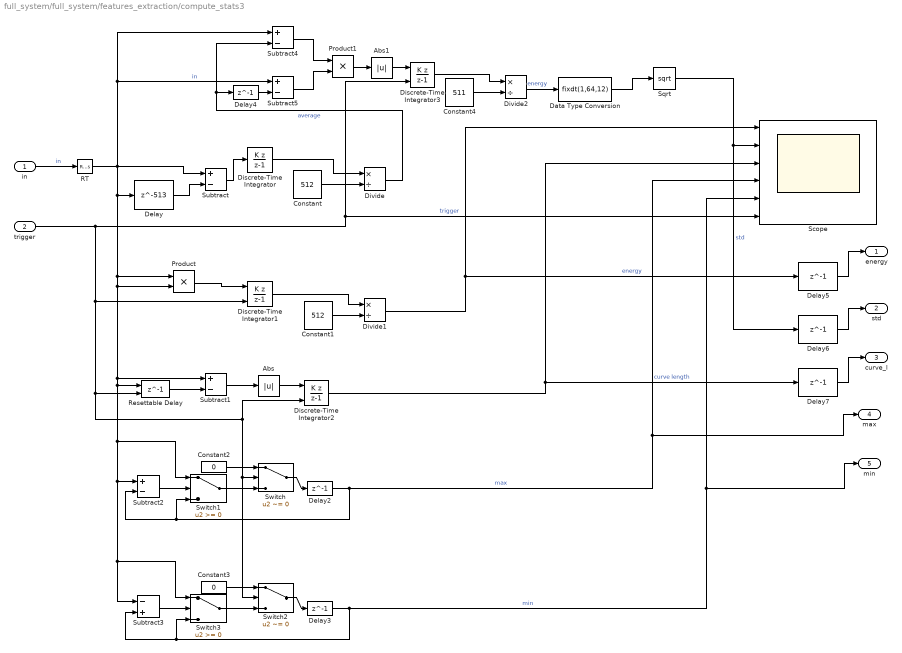
== system full_system/full_system/features_extraction/compute_stats3 ==
  in : Inport
  trigger : Inport  Port=2
  Abs : Abs
  Abs1 : Abs
  Constant : Constant  Value=512  VectorParams1D=off  OutDataTypeStr=uint16  SampleTime=-1
  Constant1 : Constant  Value=512  VectorParams1D=off  OutDataTypeStr=uint16  SampleTime=-1
  Constant2 : Constant  Value=0  VectorParams1D=off  OutDataTypeStr=uint8  SampleTime=-1
  Constant3 : Constant  Value=0  VectorParams1D=off  OutDataTypeStr=uint8  SampleTime=-1
  Constant4 : Constant  Value=511  VectorParams1D=off  OutDataTypeStr=uint16  SampleTime=-1
  Data Type Conversion : DataTypeConversion  OutMax=2  OutDataTypeStr=fixdt(1,64,12)
  Delay : Delay  DelayLength=513  InitialCondition=0  UseCircularBuffer=on
  Delay{2..7} (6 alike) : Delay  DelayLength=1  InitialCondition=0  UseCircularBuffer=on
  Discrete-Time Integrator : DiscreteIntegrator  IntegratorMethod=Accumulation: Backward Euler  SampleTime=-1  ICPrevOutput=DiscIntNeverNeededParam  ICPrevScaledInput=DiscIntNeverNeededParam
  Discrete-Time Integrator1 : DiscreteIntegrator  IntegratorMethod=Accumulation: Backward Euler  ExternalReset=rising  SampleTime=-1  ICPrevOutput=DiscIntNeverNeededParam  ICPrevScaledInput=DiscIntNeverNeededParam
  Discrete-Time Integrator2 : DiscreteIntegrator  IntegratorMethod=Accumulation: Backward Euler  ExternalReset=rising  SampleTime=-1  ICPrevOutput=DiscIntNeverNeededParam  ICPrevScaledInput=DiscIntNeverNeededParam
  Discrete-Time Integrator3 : DiscreteIntegrator  IntegratorMethod=Accumulation: Backward Euler  ExternalReset=rising  SampleTime=-1  ICPrevOutput=DiscIntNeverNeededParam  ICPrevScaledInput=DiscIntNeverNeededParam
  Divide : Product  Inputs=*/  RndMeth=Zero  SaturateOnIntegerOverflow=on  OutDataTypeStr=Inherit: Same as first input
  Divide1 : Product  Inputs=*/  RndMeth=Zero  SaturateOnIntegerOverflow=on
  Divide2 : Product  Inputs=*/  RndMeth=Zero  SaturateOnIntegerOverflow=on
  Product : Product
  Product1 : Product
  RT : RateTransition  OutPortSampleTime=1
  Resettable Delay : Delay  DelayLength=1  ExternalReset=Level
      settings: InputPortMap=u0,r5
  Scope : Scope  NumInputPorts=6
  Sqrt : Sqrt  SaturateOnIntegerOverflow=on
  Subtract{,1..2,4..5} (5 alike) : Sum  Inputs=+-
  Subtract3 : Sum  Inputs=-+
  Switch : Switch  Criteria=u2 ~= 0
  Switch1 : Switch  OutDataTypeStr=Inherit: Same as first input
  Switch2 : Switch  Criteria=u2 ~= 0
  Switch3 : Switch  OutDataTypeStr=Inherit: Same as first input
  energy : Outport
  std : Outport  Port=2
  curve_l : Outport  Port=3
  max : Outport  Port=4
  min : Outport  Port=5
  wires:
  Constant/1 -> Divide/2
  Subtract/1 -> Discrete-Time Integrator/1
  Delay/1 -> Subtract/2
  Product/1 -> Discrete-Time Integrator1/1
  Constant1/1 -> Divide1/2
  Discrete-Time Integrator1/1 -> Divide1/1
  Resettable Delay/1 -> Subtract1/2
  Subtract1/1 -> Abs/1
  Abs/1 -> Discrete-Time Integrator2/1
  Discrete-Time Integrator2/1 -> Delay7/1, Scope/3  "curve length"
  Constant2/1 -> Switch/1
  Subtract2/1 -> Switch1/2
  Delay2/1 -> max/1, Scope/4, Switch1/3, Subtract2/2  "max"
  Switch/1 -> Delay2/1
  Switch1/1 -> Switch/3
  Constant3/1 -> Switch2/1
  Switch2/1 -> Delay3/1
  Switch3/1 -> Switch2/3
  Subtract3/1 -> Switch3/2
  Delay3/1 -> min/1, Scope/5, Switch3/3, Subtract3/2  "min"
  trigger/1 -> Discrete-Time Integrator3/2, Scope/6, Discrete-Time Integrator1/2, Resettable Delay/2, Discrete-Time Integrator2/2, Switch2/2, Switch/2  "trigger"
  RT/1 -> Subtract4/1, Subtract5/1, Delay/1, Product/1, Switch1/1, Switch3/1, Subtract3/1, Subtract2/1, Resettable Delay/1, Subtract1/1, Product/2, Subtract/1  "in"
  Delay4/1 -> Subtract5/2
  Subtract4/1 -> Product1/1
  Subtract5/1 -> Product1/2
  Constant4/1 -> Divide2/2
  Discrete-Time Integrator3/1 -> Divide2/1
  Divide/1 -> Subtract4/2, Delay4/1  "average"
  Discrete-Time Integrator/1 -> Divide/1
  Divide2/1 -> Data Type Conversion/1  "energy"
  Data Type Conversion/1 -> Sqrt/1
  Product1/1 -> Abs1/1
  Abs1/1 -> Discrete-Time Integrator3/1
  Delay5/1 -> energy/1
  Delay6/1 -> std/1
  Delay7/1 -> curve_l/1
  Divide1/1 -> Scope/1, Delay5/1  "energy"
  Sqrt/1 -> Scope/2, Delay6/1  "std"
  in/1 -> RT/1  "in"

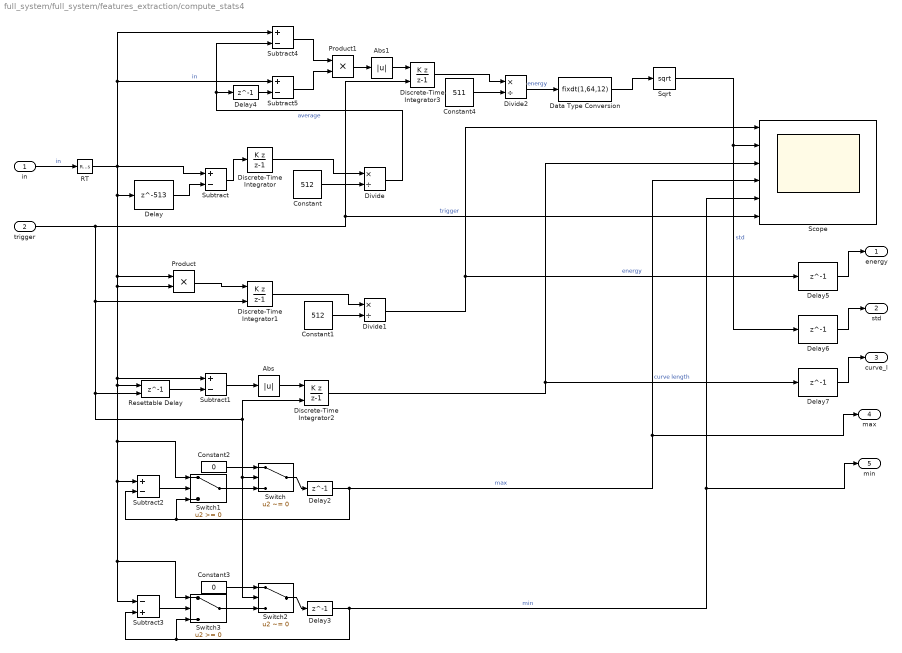
== system full_system/full_system/features_extraction/compute_stats4 ==
  in : Inport
  trigger : Inport  Port=2
  Abs : Abs
  Abs1 : Abs
  Constant : Constant  Value=512  VectorParams1D=off  OutDataTypeStr=uint16  SampleTime=-1
  Constant1 : Constant  Value=512  VectorParams1D=off  OutDataTypeStr=uint16  SampleTime=-1
  Constant2 : Constant  Value=0  VectorParams1D=off  OutDataTypeStr=uint8  SampleTime=-1
  Constant3 : Constant  Value=0  VectorParams1D=off  OutDataTypeStr=uint8  SampleTime=-1
  Constant4 : Constant  Value=511  VectorParams1D=off  OutDataTypeStr=uint16  SampleTime=-1
  Data Type Conversion : DataTypeConversion  OutMax=2  OutDataTypeStr=fixdt(1,64,12)
  Delay : Delay  DelayLength=513  InitialCondition=0  UseCircularBuffer=on
  Delay{2..7} (6 alike) : Delay  DelayLength=1  InitialCondition=0  UseCircularBuffer=on
  Discrete-Time Integrator : DiscreteIntegrator  IntegratorMethod=Accumulation: Backward Euler  SampleTime=-1  ICPrevOutput=DiscIntNeverNeededParam  ICPrevScaledInput=DiscIntNeverNeededParam
  Discrete-Time Integrator1 : DiscreteIntegrator  IntegratorMethod=Accumulation: Backward Euler  ExternalReset=rising  SampleTime=-1  ICPrevOutput=DiscIntNeverNeededParam  ICPrevScaledInput=DiscIntNeverNeededParam
  Discrete-Time Integrator2 : DiscreteIntegrator  IntegratorMethod=Accumulation: Backward Euler  ExternalReset=rising  SampleTime=-1  ICPrevOutput=DiscIntNeverNeededParam  ICPrevScaledInput=DiscIntNeverNeededParam
  Discrete-Time Integrator3 : DiscreteIntegrator  IntegratorMethod=Accumulation: Backward Euler  ExternalReset=rising  SampleTime=-1  ICPrevOutput=DiscIntNeverNeededParam  ICPrevScaledInput=DiscIntNeverNeededParam
  Divide : Product  Inputs=*/  RndMeth=Zero  SaturateOnIntegerOverflow=on  OutDataTypeStr=Inherit: Same as first input
  Divide1 : Product  Inputs=*/  RndMeth=Zero  SaturateOnIntegerOverflow=on
  Divide2 : Product  Inputs=*/  RndMeth=Zero  SaturateOnIntegerOverflow=on
  Product : Product
  Product1 : Product
  RT : RateTransition  OutPortSampleTime=1
  Resettable Delay : Delay  DelayLength=1  ExternalReset=Level
      settings: InputPortMap=u0,r5
  Scope : Scope  NumInputPorts=6
  Sqrt : Sqrt  SaturateOnIntegerOverflow=on
  Subtract{,1..2,4..5} (5 alike) : Sum  Inputs=+-
  Subtract3 : Sum  Inputs=-+
  Switch : Switch  Criteria=u2 ~= 0
  Switch1 : Switch  OutDataTypeStr=Inherit: Same as first input
  Switch2 : Switch  Criteria=u2 ~= 0
  Switch3 : Switch  OutDataTypeStr=Inherit: Same as first input
  energy : Outport
  std : Outport  Port=2
  curve_l : Outport  Port=3
  max : Outport  Port=4
  min : Outport  Port=5
  wires:
  Constant/1 -> Divide/2
  Subtract/1 -> Discrete-Time Integrator/1
  Delay/1 -> Subtract/2
  Product/1 -> Discrete-Time Integrator1/1
  Constant1/1 -> Divide1/2
  Discrete-Time Integrator1/1 -> Divide1/1
  Resettable Delay/1 -> Subtract1/2
  Subtract1/1 -> Abs/1
  Abs/1 -> Discrete-Time Integrator2/1
  Discrete-Time Integrator2/1 -> Delay7/1, Scope/3  "curve length"
  Constant2/1 -> Switch/1
  Subtract2/1 -> Switch1/2
  Delay2/1 -> max/1, Scope/4, Switch1/3, Subtract2/2  "max"
  Switch/1 -> Delay2/1
  Switch1/1 -> Switch/3
  Constant3/1 -> Switch2/1
  Switch2/1 -> Delay3/1
  Switch3/1 -> Switch2/3
  Subtract3/1 -> Switch3/2
  Delay3/1 -> min/1, Scope/5, Switch3/3, Subtract3/2  "min"
  trigger/1 -> Discrete-Time Integrator3/2, Scope/6, Discrete-Time Integrator1/2, Resettable Delay/2, Discrete-Time Integrator2/2, Switch2/2, Switch/2  "trigger"
  RT/1 -> Subtract4/1, Subtract5/1, Delay/1, Product/1, Switch1/1, Switch3/1, Subtract3/1, Subtract2/1, Resettable Delay/1, Subtract1/1, Product/2, Subtract/1  "in"
  Delay4/1 -> Subtract5/2
  Subtract4/1 -> Product1/1
  Subtract5/1 -> Product1/2
  Constant4/1 -> Divide2/2
  Discrete-Time Integrator3/1 -> Divide2/1
  Divide/1 -> Subtract4/2, Delay4/1  "average"
  Discrete-Time Integrator/1 -> Divide/1
  Divide2/1 -> Data Type Conversion/1  "energy"
  Data Type Conversion/1 -> Sqrt/1
  Product1/1 -> Abs1/1
  Abs1/1 -> Discrete-Time Integrator3/1
  Delay5/1 -> energy/1
  Delay6/1 -> std/1
  Delay7/1 -> curve_l/1
  Divide1/1 -> Scope/1, Delay5/1  "energy"
  Sqrt/1 -> Scope/2, Delay6/1  "std"
  in/1 -> RT/1  "in"

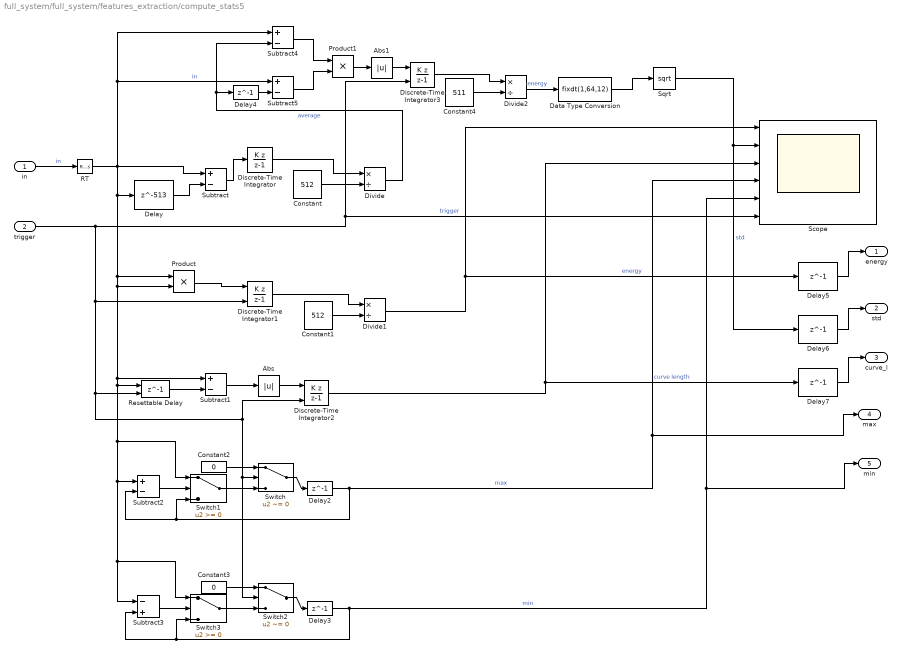
== system full_system/full_system/features_extraction/compute_stats5 ==
  in : Inport
  trigger : Inport  Port=2
  Abs : Abs
  Abs1 : Abs
  Constant : Constant  Value=512  VectorParams1D=off  OutDataTypeStr=uint16  SampleTime=-1
  Constant1 : Constant  Value=512  VectorParams1D=off  OutDataTypeStr=uint16  SampleTime=-1
  Constant2 : Constant  Value=0  VectorParams1D=off  OutDataTypeStr=uint8  SampleTime=-1
  Constant3 : Constant  Value=0  VectorParams1D=off  OutDataTypeStr=uint8  SampleTime=-1
  Constant4 : Constant  Value=511  VectorParams1D=off  OutDataTypeStr=uint16  SampleTime=-1
  Data Type Conversion : DataTypeConversion  OutMax=2  OutDataTypeStr=fixdt(1,64,12)
  Delay : Delay  DelayLength=513  InitialCondition=0  UseCircularBuffer=on
  Delay{2..7} (6 alike) : Delay  DelayLength=1  InitialCondition=0  UseCircularBuffer=on
  Discrete-Time Integrator : DiscreteIntegrator  IntegratorMethod=Accumulation: Backward Euler  SampleTime=-1  ICPrevOutput=DiscIntNeverNeededParam  ICPrevScaledInput=DiscIntNeverNeededParam
  Discrete-Time Integrator1 : DiscreteIntegrator  IntegratorMethod=Accumulation: Backward Euler  ExternalReset=rising  SampleTime=-1  ICPrevOutput=DiscIntNeverNeededParam  ICPrevScaledInput=DiscIntNeverNeededParam
  Discrete-Time Integrator2 : DiscreteIntegrator  IntegratorMethod=Accumulation: Backward Euler  ExternalReset=rising  SampleTime=-1  ICPrevOutput=DiscIntNeverNeededParam  ICPrevScaledInput=DiscIntNeverNeededParam
  Discrete-Time Integrator3 : DiscreteIntegrator  IntegratorMethod=Accumulation: Backward Euler  ExternalReset=rising  SampleTime=-1  ICPrevOutput=DiscIntNeverNeededParam  ICPrevScaledInput=DiscIntNeverNeededParam
  Divide : Product  Inputs=*/  RndMeth=Zero  SaturateOnIntegerOverflow=on  OutDataTypeStr=Inherit: Same as first input
  Divide1 : Product  Inputs=*/  RndMeth=Zero  SaturateOnIntegerOverflow=on
  Divide2 : Product  Inputs=*/  RndMeth=Zero  SaturateOnIntegerOverflow=on
  Product : Product
  Product1 : Product
  RT : RateTransition  OutPortSampleTime=1
  Resettable Delay : Delay  DelayLength=1  ExternalReset=Level
      settings: InputPortMap=u0,r5
  Scope : Scope  NumInputPorts=6
  Sqrt : Sqrt  SaturateOnIntegerOverflow=on
  Subtract{,1..2,4..5} (5 alike) : Sum  Inputs=+-
  Subtract3 : Sum  Inputs=-+
  Switch : Switch  Criteria=u2 ~= 0
  Switch1 : Switch  OutDataTypeStr=Inherit: Same as first input
  Switch2 : Switch  Criteria=u2 ~= 0
  Switch3 : Switch  OutDataTypeStr=Inherit: Same as first input
  energy : Outport
  std : Outport  Port=2
  curve_l : Outport  Port=3
  max : Outport  Port=4
  min : Outport  Port=5
  wires:
  Constant/1 -> Divide/2
  Subtract/1 -> Discrete-Time Integrator/1
  Delay/1 -> Subtract/2
  Product/1 -> Discrete-Time Integrator1/1
  Constant1/1 -> Divide1/2
  Discrete-Time Integrator1/1 -> Divide1/1
  Resettable Delay/1 -> Subtract1/2
  Subtract1/1 -> Abs/1
  Abs/1 -> Discrete-Time Integrator2/1
  Discrete-Time Integrator2/1 -> Delay7/1, Scope/3  "curve length"
  Constant2/1 -> Switch/1
  Subtract2/1 -> Switch1/2
  Delay2/1 -> max/1, Scope/4, Switch1/3, Subtract2/2  "max"
  Switch/1 -> Delay2/1
  Switch1/1 -> Switch/3
  Constant3/1 -> Switch2/1
  Switch2/1 -> Delay3/1
  Switch3/1 -> Switch2/3
  Subtract3/1 -> Switch3/2
  Delay3/1 -> min/1, Scope/5, Switch3/3, Subtract3/2  "min"
  trigger/1 -> Discrete-Time Integrator3/2, Scope/6, Discrete-Time Integrator1/2, Resettable Delay/2, Discrete-Time Integrator2/2, Switch2/2, Switch/2  "trigger"
  RT/1 -> Subtract4/1, Subtract5/1, Delay/1, Product/1, Switch1/1, Switch3/1, Subtract3/1, Subtract2/1, Resettable Delay/1, Subtract1/1, Product/2, Subtract/1  "in"
  Delay4/1 -> Subtract5/2
  Subtract4/1 -> Product1/1
  Subtract5/1 -> Product1/2
  Constant4/1 -> Divide2/2
  Discrete-Time Integrator3/1 -> Divide2/1
  Divide/1 -> Subtract4/2, Delay4/1  "average"
  Discrete-Time Integrator/1 -> Divide/1
  Divide2/1 -> Data Type Conversion/1  "energy"
  Data Type Conversion/1 -> Sqrt/1
  Product1/1 -> Abs1/1
  Abs1/1 -> Discrete-Time Integrator3/1
  Delay5/1 -> energy/1
  Delay6/1 -> std/1
  Delay7/1 -> curve_l/1
  Divide1/1 -> Scope/1, Delay5/1  "energy"
  Sqrt/1 -> Scope/2, Delay6/1  "std"
  in/1 -> RT/1  "in"
